simulink model "Tank_Modell_Student_R2013b"  (R2013a)
settings: Solver=ode45  StartTime=0.0  StopTime=400  MaxStep=1e-1  RelTol=1e-3
InitFcn:
  | set_parameter
StopFcn:
  | animation(h1_out,h2_out,q12_out,a1_out,a2_out,z1_out,anim_on,video_on);
values from neighbouring files (symbols this model uses):
  parInit =     [parameter_08.mat]
  parSys =     [parameter_08.mat]
undefined symbols (not defined in the file or in its folder): parSollwertfilter
libraries: simulink x3
settings Model: Creator=Wolfgang Kemmetmüller  LastModifiedBy=Christoph Zech
settings DataIOCC: SignalLoggingSaveFormat=ModelDataLogs
settings OptimizationCC: ExpressionDepthLimit=2147483647  InitFltsAndDblsToZero=on
settings DebuggingCC: SaveWithParameterizedLinksMsg=none  MultiTaskDSMMsg=warning  MultiTaskCondExecSysMsg=none  FrameProcessingCompatibilityMsg=error  StrictBusMsg=None
settings SFSimCC: SimParseCustomCode=off
settings RTWCC: IncludeERTFirstTime=on
settings GRTTargetCC: CodeReplacementLibrary=C89/C90 (ANSI)  CombineOutputUpdateFcns=off  GRTInterface=on

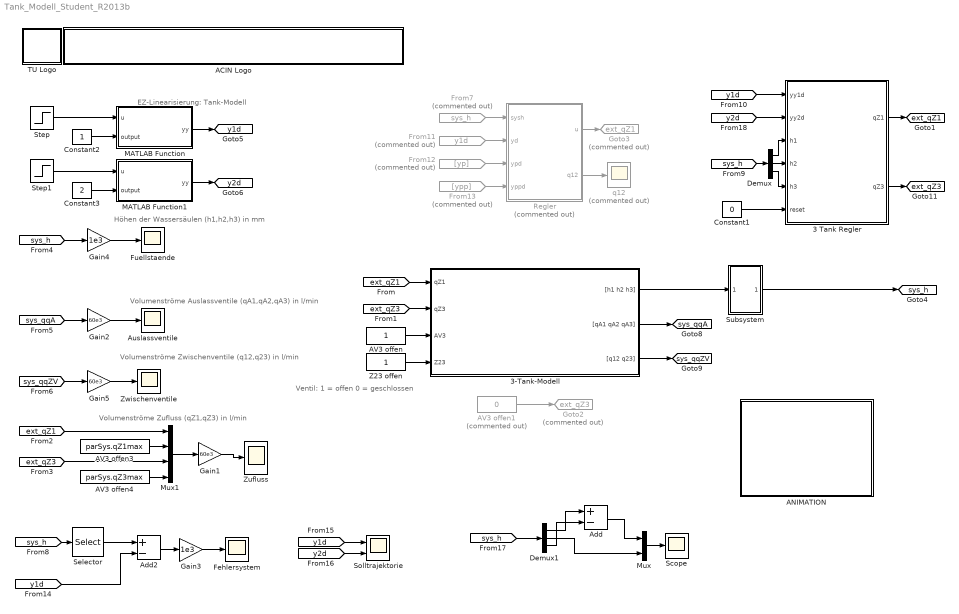
== system Tank_Modell_Student_R2013b ==
  note: EZ-Linearisierung: Tank-Modell
  note: Höhen der Wassersäulen (h1,h2,h3) in mm
  note: Volumenströme Auslassventile (qA1,qA2,qA3) in l/min
  note: Volumenströme Zwischenventile (q12,q23) in l/min
  note: Ventil:
      | 1 = offen
      | 0 = geschlossen
  note: Volumenströme Zufluss (qZ1,qZ3) in l/min
  3 Tank Regler : MATLAB Function  TreatAsAtomicUnit=on
  3-Tank-Modell : Subsystem
      mask init:
      | S = get_param(gcb,'UserData');
      mask Display:
      | image(S.pic);
      | port_label('input', 1, 'qZ1');
      | port_label('input', 2, 'qZ3');
      | port_label('input', 3, 'AV3');
      | port_label('input', 4, 'Z23');
      | port_label('output', 1, '[h1 h2 h3]');
      | port_label('output', 2, '[qA1 qA2 qA3]');
      | port_label('output', 3, '[q12 q23]');
  ACIN Logo : Subsystem
      mask init:
      | s = get_param(gcb,'UserData');
      mask Display:
      | image(s.logo,[0 0 439 45]);
      | %axis image
  ANIMATION : Subsystem
      mask init:
      | S = get_param(gcb,'UserData');
      mask Display: image(imread('Fisch.jpg'));
  AV3 offen : Constant
  AV3 offen1 : Constant  Commented=on  Value=0
  AV3 offen3 : Constant  Value=parSys.qZ1max  SampleTime=parSys.Ta
  AV3 offen4 : Constant  Value=parSys.qZ3max  SampleTime=parSys.Ta
  Add : Sum  Inputs=+-
  Add2 : Sum  Inputs=+-
  Auslassventile : Scope
      settings: ShowLegends=on  YMin=0.56181  YMax=1.40614
  Constant1 : Constant  Value=0
  Constant2 : Constant
  Constant3 : Constant  Value=2
  Demux : Demux  Outputs=3
  Demux1 : Demux  Outputs=3
  Fehlersystem : Scope
      settings: ShowLegends=on  YMin=-10  YMax=140  SaveName=ScopeData2
  From11 : From  Commented=on  GotoTag=y1d  TagVisibility=global
  From12 : From  Commented=on  GotoTag=yp  TagVisibility=global
  From13 : From  Commented=on  GotoTag=ypp  TagVisibility=global
  From7 : From  Commented=on  GotoTag=sys_h  TagVisibility=global
  Fuellstaende : Scope
      settings: ShowLegends=on  YMin=90  YMax=250
  Gain1 : Gain  Gain=60e3
  Gain2 : Gain  Gain=60e3
  Gain3 : Gain  Gain=1e3
  Gain4 : Gain  Gain=1e3
  Gain5 : Gain  Gain=60e3
  Goto2 : Goto  Commented=on  GotoTag=ext_qZ3  TagVisibility=global
  Goto3 : Goto  Commented=on  GotoTag=ext_qZ1  TagVisibility=global
  MATLAB Function : MATLAB Function  TreatAsAtomicUnit=on  SystemSampleTime=parSollwertfilter.Ta
  MATLAB Function1 : MATLAB Function  TreatAsAtomicUnit=on  SystemSampleTime=parSollwertfilter.Ta
  Mux : Mux  Inputs=2
  Mux1 : Mux
  "Regler " : MATLAB Function  Commented=on  TreatAsAtomicUnit=on
  Scope : Scope
      settings: YMin=0.03  YMax=0.21  SaveName=ScopeData5
  Selector : Selector  InputPortWidth=3  IndexOptions=Index vector (dialog)  Indices=[2]  OutputSizes=1
  Solltrajektorie : Scope  NumInputPorts=2
      settings: YMin=-0.0125~-0.0125  YMax=0.1125~0.1125
  Step : Step  Before=parSys.h2_0  After=parSys.h2_0+0.1  SampleTime=0
  Step1 : Step  Before=parSys.h1_0-parSys.h3_0  After=parSys.h1_0-parSys.h3_0-0.05  SampleTime=0
  Subsystem : Subsystem
  TU Logo : Subsystem
      mask init:
      | s = get_param(gcb,'UserData');
      mask Display: image(s.logo,[0 0 45 45]);
  Z23 offen : Constant
  Zufluss : Scope
      settings: ShowLegends=on  YMin=-7.5  YMax=22.5  SaveName=ScopeData3
  Zwischenventile : Scope
      settings: YMin=-10  YMax=10  SaveName=ScopeData2
  q12 : Scope  Commented=on
      settings: ShowLegends=on  YMin=0.000014  YMax=0.000028  SaveName=ScopeData4
  tag scope: ext_qZ1=global, ext_qZ3=global, sys_h=global, sys_qqA=global, sys_qqZV=global, y1d=global, y2d=global
  wires:
  [sys_qqA] -> Gain2/1
  [sys_qqZV] -> Gain5/1
  [sys_h] -> Gain4/1
  3-Tank-Modell/3("[q12 q23]") -> [sys_qqZV]
  3-Tank-Modell/2("[qA1 qA2 qA3]") -> [sys_qqA]
  AV3 offen/1 -> 3-Tank-Modell/3(AV3)
  Z23 offen/1 -> 3-Tank-Modell/4(Z23)
  [ext_qZ1] -> 3-Tank-Modell/1(qZ1)
  [ext_qZ3] -> 3-Tank-Modell/2(qZ3)
  [ext_qZ1] -> Mux1/1
  [ext_qZ3] -> Mux1/3
  AV3 offen3/1 -> Mux1/2
  AV3 offen4/1 -> Mux1/4
  Gain5/1 -> Zwischenventile/1
  Gain2/1 -> Auslassventile/1
  Gain4/1 -> Fuellstaende/1
  Mux1/1 -> Gain1/1
  Gain1/1 -> Zufluss/1
  AV3 offen1/1 -> Goto2/1
  "Regler "/1(u) -> Goto3/1
  From7/1 -> "Regler "/1(sysh)
  [sys_h] -> Selector/1
  Selector/1 -> Add2/1
  "Regler "/2(q12) -> q12/1
  MATLAB Function/1(yy) -> [y1d]
  From11/1 -> "Regler "/2(yd)
  From12/1 -> "Regler "/3(ypd)
  From13/1 -> "Regler "/4(yppd)
  [y1d] -> Add2/2
  [y1d] -> Solltrajektorie/1
  [y2d] -> Solltrajektorie/2
  Add2/1 -> Gain3/1
  Gain3/1 -> Fehlersystem/1
  [sys_h] -> Demux/1
  Demux/1 -> 3 Tank Regler/3(h1)
  Demux/2 -> 3 Tank Regler/4(h2)
  Demux/3 -> 3 Tank Regler/5(h3)
  3 Tank Regler/1(qZ1) -> [ext_qZ1]
  3 Tank Regler/2(qZ3) -> [ext_qZ3]
  Constant1/1 -> 3 Tank Regler/6(reset)
  [y1d] -> 3 Tank Regler/1(yy1d)
  Constant2/1 -> MATLAB Function/2(output)
  MATLAB Function1/1(yy) -> [y2d]
  Constant3/1 -> MATLAB Function1/2(output)
  [y2d] -> 3 Tank Regler/2(yy2d)
  Step/1 -> MATLAB Function/1(u)
  Step1/1 -> MATLAB Function1/1(u)
  [sys_h] -> Demux1/1
  Demux1/1 -> Add/1
  Demux1/3 -> Add/2
  Mux/1 -> Scope/1
  Add/1 -> Mux/1
  Demux1/2 -> Mux/2
  3-Tank-Modell/1("[h1 h2 h3]") -> Subsystem/1(In1)
  Subsystem/1(Out1) -> [sys_h]

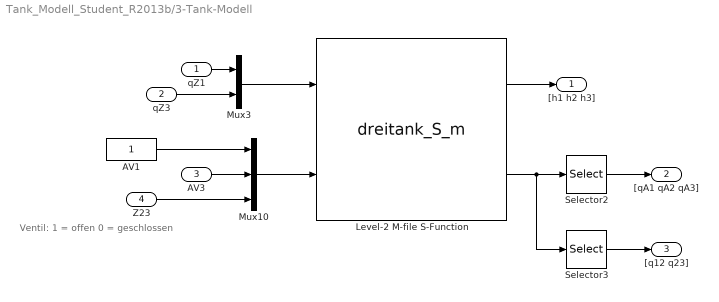
== system Tank_Modell_Student_R2013b/3-Tank-Modell ==
  note: Ventil:
      | 1 = offen
      | 0 = geschlossen
  qZ1 : Inport
  qZ3 : Inport  Port=2
  AV3 : Inport  Port=3
  Z23 : Inport  Port=4
  AV1 : Constant
  Level-2 M-file S-Function : M-S-Function  FunctionName=dreitank_S_m  Parameters=Atank, rho, eta, g, alphaA1, DA1, alphaA2, A2, alphaA3, DA3, alpha12_0, A12, Dh12, lambdac12, alpha23_0, D23, lambdac23, hmin, h1_0, h2_0, h3_0, qZ1max, qZ3max, flaglimqZ, h_max, h_min  mask{Atank=parSys.Atank, rho=parSys.rho, eta=parSys.eta, g=parSys.g, alphaA1=parSys.alphaA1, DA1=parSys.DA1, alphaA2=parSys.alphaA2, A2=parSys.A2, alphaA3=parSys.alphaA3, DA3=parSys.DA3, alpha12_0=parSys.alpha12_0, A12=parSys.A12, Dh12=parSys.Dh12, lambdac12=parSys.lambdac12, alpha23_0=parSys.alpha23_0, D23=parSys.D23, lambdac23=parSys.lambdac23, hmin=parSys.hmin, h1_0=parSys.h1_0, h2_0=parSys.h2_0, h3_0=parSys.h3_0, qZ1max=parSys.qZ1max, qZ3max=parSys.qZ3max, h_max=parSys.hmax, h_min=parSys.hmin, flaglimqZ=off}
      mask prompts: Atank "Grundfläche Tank (Atank)"; rho "Dichte Wasser (rho)"; eta "Viskosität Wasser (eta)"; g "Gravitationskonstante (g)"; alphaA1 "Kontraktionskoeffizient AV1 (alphaA1)"; DA1 "Durchmesser AV1 (DA1)"; alphaA2 "Kontraktionskoeffizient AV2 (alphaA2)"; A2 "Querschnittsfläche AV2 (A2)"; alphaA3 "Kontraktionskoeffizient AV3 (alphaA3)"; DA3 "Durchmesser A3 (DA3)"; alpha12_0 "Kontraktionskoeffizient ZV12 (alpha12_0)"; A12 "Querschnittsfläche ZV12 (A12)"; Dh12 "hydraulischer Durchmesser ZV12 (Dh12)"; lambdac12 "kritische Fließzahl ZV12 (lambdac12)"; alpha23_0 "Kontraktionskoeffizient ZV23 (alpha23_0)"; D23 "Durchmesser ZV23 (D23)"; lambdac23 "kritische Fließzahl ZV23 (lambdac23)"; hmin "minimale Füllhöhe (hmin)"; h1_0 "Anfangsbedingung h1 (h1_0)"; h2_0 "Anfangsbedingung h2 (h2_0)"; h3_0 "Anfangsbedingung h3 (h3_0)"; qZ1max "maximaler Zufluss Z1 (qZ1max)"; qZ3max "maximaler Zufluss Z3 (qZ3max)"; h_max "Maximale Füllhöhe"; h_min "Minimale Füllhöhe"; flaglimqZ "Beschränkung der Zuflüsse ein"
      mask Display:
      | port_label('input',1,'Zulaufvolumenströme')
      | port_label('input',2,'Zustand Ventile')
      | 
      | port_label('output',1,'Zustände')
      | port_label('output',2,'Volumenströme')
  Mux10 : Mux  Inputs=3
  Mux3 : Mux  Inputs=2
  Selector2 : Selector  InputPortWidth=5  IndexOptions=Index vector (dialog)  Indices=[1 2 3]  OutputSizes=1
  Selector3 : Selector  InputPortWidth=5  IndexOptions=Index vector (dialog)  Indices=[4 5]  OutputSizes=1
  "[h1 h2 h3]" : Outport
  "[qA1 qA2 qA3]" : Outport  Port=2
  "[q12 q23]" : Outport  Port=3
  wires:
  AV1/1 -> Mux10/1
  Mux3/1 -> Level-2 M-file S-Function/1
  Mux10/1 -> Level-2 M-file S-Function/2
  qZ1/1 -> Mux3/1
  Level-2 M-file S-Function/1 -> "[h1 h2 h3]"/1
  qZ3/1 -> Mux3/2
  Level-2 M-file S-Function/2 -> Selector2/1, Selector3/1
  Selector2/1 -> "[qA1 qA2 qA3]"/1
  Selector3/1 -> "[q12 q23]"/1
  Z23/1 -> Mux10/3
  AV3/1 -> Mux10/2

== system Tank_Modell_Student_R2013b/ACIN Logo ==

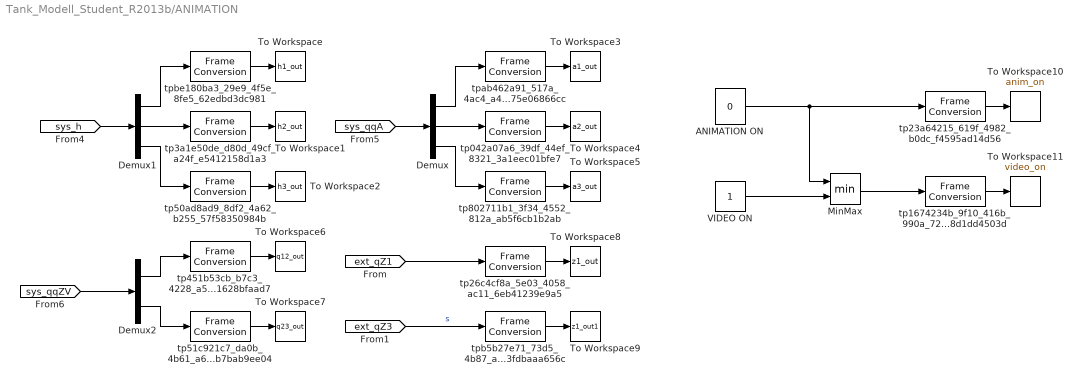
== system Tank_Modell_Student_R2013b/ANIMATION ==
  ANIMATION ON : Constant  Value=0
  Demux : Demux  Outputs=3
  Demux1 : Demux  Outputs=3
  Demux2 : Demux  Outputs=2
  MinMax : MinMax  Inputs=2
  To Workspace : ToWorkspace  VariableName=h1_out  SampleTime=parSys.Ta
  To Workspace1 : ToWorkspace  VariableName=h2_out  SampleTime=parSys.Ta
  To Workspace10 : ToWorkspace  VariableName=anim_on  SampleTime=50
  To Workspace11 : ToWorkspace  VariableName=video_on  SampleTime=50
  To Workspace2 : ToWorkspace  VariableName=h3_out  SampleTime=parSys.Ta
  To Workspace3 : ToWorkspace  VariableName=a1_out  SampleTime=parSys.Ta
  To Workspace4 : ToWorkspace  VariableName=a2_out  SampleTime=parSys.Ta
  To Workspace5 : ToWorkspace  VariableName=a3_out  SampleTime=parSys.Ta
  To Workspace6 : ToWorkspace  VariableName=q12_out  SampleTime=parSys.Ta
  To Workspace7 : ToWorkspace  VariableName=q23_out  SampleTime=parSys.Ta
  To Workspace8 : ToWorkspace  VariableName=z1_out  SampleTime=parSys.Ta
  To Workspace9 : ToWorkspace  VariableName=z1_out1  SampleTime=parSys.Ta
  VIDEO ON : Constant
  tp042a07a6_39df_44ef_8321_3a1eec01bfe7 : FrameConversion  OutFrame=Sample-based
  tp1674234b_9f10_416b_990a_728d1dd4503d : FrameConversion  OutFrame=Sample-based
  tp23a64215_619f_4982_b0dc_f4595ad14d56 : FrameConversion  OutFrame=Sample-based
  tp26c4cf8a_5e03_4058_ac11_6eb41239e9a5 : FrameConversion  OutFrame=Sample-based
  tp3a1e50de_d80d_49cf_a24f_e5412158d1a3 : FrameConversion  OutFrame=Sample-based
  tp451b53cb_b7c3_4228_a556_c61628bfaad7 : FrameConversion  OutFrame=Sample-based
  tp50ad8ad9_8df2_4a62_b255_57f58350984b : FrameConversion  OutFrame=Sample-based
  tp51c921c7_da0b_4b61_a6ab_b6b7bab9ee04 : FrameConversion  OutFrame=Sample-based
  tp802711b1_3f34_4552_812a_ab5f6cb1b2ab : FrameConversion  OutFrame=Sample-based
  tpab462a91_517a_4ac4_a466_6d75e06866cc : FrameConversion  OutFrame=Sample-based
  tpb5b27e71_73d5_4b87_ab88_53fdbaaa656c : FrameConversion  OutFrame=Sample-based
  tpbe180ba3_29e9_4f5e_8fe5_62edbd3dc981 : FrameConversion  OutFrame=Sample-based
  wires:
  [sys_qqA] -> Demux/1
  [sys_h] -> Demux1/1
  [sys_qqZV] -> Demux2/1
  ANIMATION ON/1 -> MinMax/1, tp23a64215_619f_4982_b0dc_f4595ad14d56/1
  VIDEO ON/1 -> MinMax/2
  Demux1/1 -> tpbe180ba3_29e9_4f5e_8fe5_62edbd3dc981/1
  tpbe180ba3_29e9_4f5e_8fe5_62edbd3dc981/1 -> To Workspace/1
  Demux1/2 -> tp3a1e50de_d80d_49cf_a24f_e5412158d1a3/1
  tp3a1e50de_d80d_49cf_a24f_e5412158d1a3/1 -> To Workspace1/1
  tp23a64215_619f_4982_b0dc_f4595ad14d56/1 -> To Workspace10/1
  MinMax/1 -> tp1674234b_9f10_416b_990a_728d1dd4503d/1
  tp1674234b_9f10_416b_990a_728d1dd4503d/1 -> To Workspace11/1
  Demux1/3 -> tp50ad8ad9_8df2_4a62_b255_57f58350984b/1
  tp50ad8ad9_8df2_4a62_b255_57f58350984b/1 -> To Workspace2/1
  Demux/1 -> tpab462a91_517a_4ac4_a466_6d75e06866cc/1
  tpab462a91_517a_4ac4_a466_6d75e06866cc/1 -> To Workspace3/1
  Demux/2 -> tp042a07a6_39df_44ef_8321_3a1eec01bfe7/1
  tp042a07a6_39df_44ef_8321_3a1eec01bfe7/1 -> To Workspace4/1
  Demux/3 -> tp802711b1_3f34_4552_812a_ab5f6cb1b2ab/1
  tp802711b1_3f34_4552_812a_ab5f6cb1b2ab/1 -> To Workspace5/1
  Demux2/1 -> tp451b53cb_b7c3_4228_a556_c61628bfaad7/1
  tp451b53cb_b7c3_4228_a556_c61628bfaad7/1 -> To Workspace6/1
  Demux2/2 -> tp51c921c7_da0b_4b61_a6ab_b6b7bab9ee04/1
  tp51c921c7_da0b_4b61_a6ab_b6b7bab9ee04/1 -> To Workspace7/1
  [ext_qZ1] -> tp26c4cf8a_5e03_4058_ac11_6eb41239e9a5/1
  tp26c4cf8a_5e03_4058_ac11_6eb41239e9a5/1 -> To Workspace8/1
  [ext_qZ3] -> tpb5b27e71_73d5_4b87_ab88_53fdbaaa656c/1  "s"
  tpb5b27e71_73d5_4b87_ab88_53fdbaaa656c/1 -> To Workspace9/1

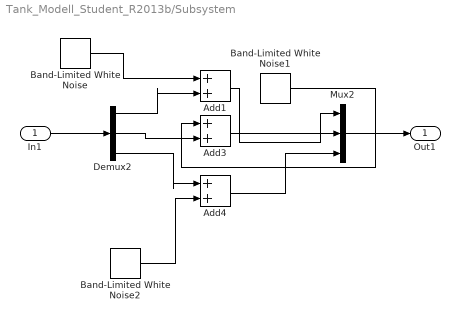
== system Tank_Modell_Student_R2013b/Subsystem ==
  In1 : Inport
  Add1 : Sum
  Add3 : Sum
  Add4 : Sum
  Band-Limited White Noise : simulink/Sources/Band-Limited White Noise  Cov=[25e-10]  Ts=0.1  seed=[23341]
  Band-Limited White Noise1 : simulink/Sources/Band-Limited White Noise  Cov=[25e-10]  Ts=0.1  seed=[93754]
  Band-Limited White Noise2 : simulink/Sources/Band-Limited White Noise  Cov=[25e-10]  Ts=0.1  seed=[35936]
  Demux2 : Demux  Outputs=3
  Mux2 : Mux  Inputs=3
  Out1 : Outport
  wires:
  Mux2/1 -> Out1/1
  In1/1 -> Demux2/1
  Add4/1 -> Mux2/3
  Demux2/2 -> Add3/2
  Band-Limited White Noise2/1 -> Add4/2
  Band-Limited White Noise1/1 -> Add3/1
  Demux2/3 -> Add4/1
  Demux2/1 -> Add1/2
  Band-Limited White Noise/1 -> Add1/1
  Add1/1 -> Mux2/1
  Add3/1 -> Mux2/2

== system Tank_Modell_Student_R2013b/TU Logo ==

== matlab function Tank_Modell_Student_R2013b/MATLAB Function ==
  settings: updateMethod=DISCRETE  sampleTime=parSollwertfilter.Ta
  data: u input; output input; yy output; parSollwertfilter parameter; parSys parameter
function yy  = sollwertfilter(u, output, parSollwertfilter, parSys)
persistent x;

if output < 1.5
    u = u-parSys.h2_0; % Anfangswert abziehen
else
    u = u-parSys.h1_0+parSys.h3_0;
end

a=parSollwertfilter.a;
b=parSollwertfilter.b;
c=parSollwertfilter.c;
d=parSollwertfilter.d;

if(isempty(x))
    x0_Filter=parSollwertfilter.x0_Filter;
    x=x0_Filter;
end

yt=c*x+d*u;

if output < 1.5
    y=yt(1)+parSys.h2_0; % Anfangswert wieder addieren
else
    y=yt(1)+parSys.h1_0-parSys.h3_0; % Anfangswert wieder addieren
end
yp=yt(2);
ypp=yt(3);

yy = [y; yp; ypp];

x=a*x+b*u;

== matlab function Tank_Modell_Student_R2013b/Regler  ==
  settings: updateMethod=DISCRETE  sampleTime=parSys.Ta
  data: u output; sysh input; parSys parameter; yd input; ypd input; yppd input; q12 output
function [u,q12]  = fcn(sysh, parSys, yd, ypd, yppd)

Atank = parSys.Atank;
rho = parSys.rho;
eta = parSys.eta;
g = parSys.g;
alphaA1 = parSys.alphaA1;
DA1 = parSys.DA1;
alphaA2 = parSys.alphaA2;
A2 = parSys.A2;
alphaA3 = parSys.alphaA3;
DA3 = parSys.DA3;
alpha12_0 = parSys.alpha12_0;
A12 = parSys.A12;
Dh12 = parSys.Dh12;
lambdac12 = parSys.lambdac12;
alpha23_0 = parSys.alpha23_0;
D23 = parSys.D23;
lambdac23 = parSys.lambdac23;
hmin = parSys.hmin;
hmax = parSys.hmax;
dh12min = parSys.dh12min;
a0 = parSys.a0;
a1 = parSys.a1;

h1=sysh(1);
h2=sysh(2);
qA1 = alphaA1 * DA1 ^ 2 * pi * sqrt(0.2e1) * sqrt(g) * sqrt(h1) / 0.4e1;
qA2 = alphaA2 * A2 * sqrt(0.2e1) * sqrt(g) * sqrt(h2);

dqA2_dh2 = alphaA2 * A2 * sqrt(0.2e1) * sqrt(g) * h2 ^ (-0.1e1 / 0.2e1) / 0.2e1;

if abs(h1-h2) > dh12min
    dq12_dh1 = 0.2e1 * alpha12_0 * Dh12 * rho / eta * g / lambdac12 * (0.1e1 - tanh(0.2e1 * Dh12 * rho / eta * sqrt(0.2e1) * sqrt(g) * sqrt(abs(h1 - h2)) / lambdac12) ^ 2) * A12 + alpha12_0 * tanh(0.2e1 * Dh12 * rho / eta * sqrt(0.2e1) * sqrt(g) * sqrt(abs(h1 - h2)) / lambdac12) * A12 * sqrt(0.2e1) * sqrt(g) * (abs(h1 - h2) ^ (-0.1e1 / 0.2e1)) / 0.2e1;
    dq12_dh2 = -0.2e1 * alpha12_0 * Dh12 * rho / eta * g / lambdac12 * (0.1e1 - tanh(0.2e1 * Dh12 * rho / eta * sqrt(0.2e1) * sqrt(g) * sqrt(abs(h1 - h2)) / lambdac12) ^ 2) * A12 - alpha12_0 * tanh(0.2e1 * Dh12 * rho / eta * sqrt(0.2e1) * sqrt(g) * sqrt(abs(h1 - h2)) / lambdac12) * A12 * sqrt(0.2e1) * sqrt(g) * (abs(h1 - h2) ^ (-0.1e1 / 0.2e1)) / 0.2e1;
else
    %Linearisierung
    dq12_dh1 = parSys.d_dh1 + parSys.k_dh1*abs(h1-h2);
    dq12_dh2 = parSys.d_dh2 + parSys.k_dh2*abs(h1-h2);
end
q12 = alpha12_0 * tanh(0.2e1 * Dh12 * rho / eta * sqrt(0.2e1) * sqrt(g) * sqrt(abs(h1 - h2)) / lambdac12) * A12 * sqrt(0.2e1) * sqrt(g) * sqrt(abs(h1 - h2)) * sign((h1 - h2));

u = 0.1e1 / dq12_dh1 * Atank ^ 2 * (yppd - dq12_dh1 / Atank ^ 2 * (-q12 - qA1) - (dq12_dh2 - dqA2_dh2) / Atank ^ 2 * (q12 - qA2) - a0 * (h2 - yd) - a1 * ((q12 - qA2) / Atank - ypd));

== matlab function Tank_Modell_Student_R2013b/3 Tank Regler ==
  settings: updateMethod=DISCRETE  sampleTime=parSys.Ta
  data: qZ1 output; qZ3 output; yy1d input; yy2d input; h1 input; h2 input; h3 input; reset input; parSys parameter; parInit parameter
function [qZ1,qZ3]  = fcn(yy1d, yy2d, h1, h2, h3, reset, parSys, parInit)

persistent e1I;
persistent e2I;

if (isempty(e1I))
    e1I = 0;
end
if (isempty(e2I))
    e2I = 0;
end
if reset
    qZ1 = 0;
    qZ3 = 0;
    return
end
    

Atank = parSys.Atank;
rho = parSys.rho;
eta = parSys.eta;
g = parSys.g;
alphaA1 = parSys.alphaA1;
DA1 = parSys.DA1;
alphaA2 = parSys.alphaA2;
A2 = parSys.A2;
alphaA3 = parSys.alphaA3;
DA3 = parSys.DA3;
alpha12_0 = parSys.alpha12_0;
A12 = parSys.A12;
Dh12 = parSys.Dh12;
lambdac12 = parSys.lambdac12;
alpha23_0 = parSys.alpha23_0;
D23 = parSys.D23;
lambdac23 = parSys.lambdac23;
hmin = parSys.hmin;
hmax = parSys.hmax;
dh12min = parSys.dh12min;
a0 = parInit.a0;
a1 = parInit.a1;
dh23min = parSys.dh12min;

A3 = DA3^2*pi/4;
%laut angabe
Dh23 = D23;
A23 = D23^2*pi/4;

y1dpp = yy1d(3);
y1dp  = yy1d(2);
y1d   = yy1d(1);

y2dp  = yy2d(2);
y2d   = yy2d(1);


qA1 = alphaA1 * DA1 ^ 2 * pi * sqrt(0.2e1) * sqrt(g) * sqrt(h1) / 0.4e1;
qA2 = alphaA2 * A2 * sqrt(0.2e1) * sqrt(g) * sqrt(h2);
qA3 = alphaA3 * A3 * sqrt(0.2e1) * sqrt(g) * sqrt(h3);


dqA2_dh2 = alphaA2 * A2 * sqrt(0.2e1) * sqrt(g) * h2 ^ (-0.1e1 / 0.2e1) / 0.2e1;

if abs(h1-h2) > dh12min
    dq12_dh1 = 0.2e1 * alpha12_0 * Dh12 * rho / eta * g / lambdac12 * (0.1e1 - tanh(0.2e1 * Dh12 * rho / eta * sqrt(0.2e1) * sqrt(g) * sqrt(abs(h1 - h2)) / lambdac12) ^ 2) * A12 + alpha12_0 * tanh(0.2e1 * Dh12 * rho / eta * sqrt(0.2e1) * sqrt(g) * sqrt(abs(h1 - h2)) / lambdac12) * A12 * sqrt(0.2e1) * sqrt(g) * (abs(h1 - h2) ^ (-0.1e1 / 0.2e1)) / 0.2e1;
    dq12_dh2 = -0.2e1 * alpha12_0 * Dh12 * rho / eta * g / lambdac12 * (0.1e1 - tanh(0.2e1 * Dh12 * rho / eta * sqrt(0.2e1) * sqrt(g) * sqrt(abs(h1 - h2)) / lambdac12) ^ 2) * A12 - alpha12_0 * tanh(0.2e1 * Dh12 * rho / eta * sqrt(0.2e1) * sqrt(g) * sqrt(abs(h1 - h2)) / lambdac12) * A12 * sqrt(0.2e1) * sqrt(g) * (abs(h1 - h2) ^ (-0.1e1 / 0.2e1)) / 0.2e1;
else
    %Linearisierung
    dq12_dh1 = parSys.d_dq12_dh1 + parSys.k_dq12_dh1*abs(h1-h2);
    dq12_dh2 = parSys.d_dq12_dh2 + parSys.k_dq12_dh2*abs(h1-h2);
end

if abs(h2-h3) > dh23min
    dq23_dh2 = 0.2e1 * alpha23_0 * (0.1e1 - tanh(0.2e1 * Dh23 * rho / eta * sqrt(0.2e1) * sqrt(g) * sqrt(abs(h2 - h3)) / lambdac23) ^ 2) * Dh23 * rho / eta * g / lambdac23 * A23 + alpha23_0 * tanh(0.2e1 * Dh23 * rho / eta * sqrt(0.2e1) * sqrt(g) * sqrt(abs(h2 - h3)) / lambdac23) * A23 * sqrt(0.2e1) * sqrt(g) * (abs(h2 - h3)) ^ (-0.1e1 / 0.2e1) / 0.2e1;
    %dq23_dh3 = 0.2e1 * alpha23_0 * (0.1e1 - tanh(0.2e1 * Dh23 * rho / eta * sqrt(0.2e1) * sqrt(g) * sqrt(abs(h3 - h2)) / lambdac23) ^ 2) * Dh23 * rho / eta * g / lambdac23 * A23 + alpha23_0 * tanh(0.2e1 * Dh23 * rho / eta * sqrt(0.2e1) * sqrt(g) * sqrt(abs(h3 - h2)) / lambdac23) * A23 * sqrt(0.2e1) * sqrt(g) * (abs(h3 - h2)) ^ (-0.1e1 / 0.2e1) / 0.2e1;
    %dq23_dh3 = 0.2e1 * alpha23_0 * (0.1e1 - tanh(0.2e1 * Dh23 * rho / eta * sqrt(0.2e1) * sqrt(g) * sqrt(abs(h3 - h2)) / lambdac23) ^ 2) * Dh23 * rho / eta * g / lambdac23 * A23 - alpha23_0 * tanh(0.2e1 * Dh23 * rho / eta * sqrt(0.2e1) * sqrt(g) * sqrt(abs(h3 - h2)) / lambdac23) * A23 * sqrt(0.2e1) * sqrt(g) * (abs(h3 - h2)) ^ (-0.1e1 / 0.2e1) / 0.2e1;
    dq23_dh3 = -0.2e1 * alpha23_0 * (0.1e1 - tanh(0.2e1 * Dh23 * rho / eta * sqrt(0.2e1) * sqrt(g) * sqrt(abs(h2 - h3)) / lambdac23) ^ 2) * Dh23 * rho / eta * g / lambdac23 * A23 - alpha23_0 * tanh(0.2e1 * Dh23 * rho / eta * sqrt(0.2e1) * sqrt(g) * sqrt(abs(h2 - h3)) / lambdac23) * A23 * sqrt(0.2e1) * sqrt(g) * abs(h2 - h3) ^ (-0.1e1 / 0.2e1) / 0.2e1;
else
    %Linearisierung
    dq23_dh2 = parSys.d_dq23_dh2 + parSys.k_dq23_dh2*abs(h2-h3);
    dq23_dh3 = parSys.d_dq23_dh3 + parSys.k_dq23_dh3*abs(h2-h3);
end

q12 = alpha12_0 * tanh(0.2e1 * Dh12 * rho / eta * sqrt(0.2e1) * sqrt(g) * sqrt(abs(h1 - h2)) / lambdac12) * A12 * sqrt(0.2e1) * sqrt(g) * sqrt(abs(h1 - h2)) * sign((h1 - h2));
q23 = alpha23_0 * tanh(0.2e1 * Dh23 * rho / eta * sqrt(0.2e1) * sqrt(g) * sqrt(abs(h2 - h3)) / lambdac23) * A23 * sqrt(0.2e1) * sqrt(g) * sqrt(abs(h2 - h3)) * sign(h2 - h3);

Lfh1 = [(q12 - q23 - qA2) / Atank];
Lf2h1 = [dq12_dh1 / Atank ^ 2 * (-q12 - qA1) - dq23_dh2 / Atank ^ 2 * (q12 - q23 - qA2) - dq23_dh3 / Atank ^ 2 * (q23 - qA3)];
Lfh2 = [(-q12 - qA1) / Atank - (q23 - qA3) / Atank];
Lg2h2 = [-0.1e1 / Atank];
Lg1h2 = [0.1e1 / Atank];
Lg2Lf1h1 = [-dq23_dh3 / Atank ^ 2];
Lg1Lf1h1 = [dq12_dh1 / Atank ^ 2];


e1I = e1I + (h2-y1d);
e2I = e2I + (h1-h3-y2d);
v = [y1dpp - parInit.a10 * (h2 - y1d) - parInit.a11 * (Lfh1 - y1dp) - parInit.a1I*e1I;
     y2dp  - parInit.a20 * (h1 - h3 - y2d) - parInit.a2I*e2I
     ];

bb = [Lf2h1;Lfh2];
D_inv = [-Lg2h2 / (Lg1h2 * Lg2Lf1h1 - Lg2h2 * Lg1Lf1h1) Lg2Lf1h1 / (Lg1h2 * Lg2Lf1h1 - Lg2h2 * Lg1Lf1h1); Lg1h2 / (Lg1h2 * Lg2Lf1h1 - Lg2h2 * Lg1Lf1h1) -Lg1Lf1h1 / (Lg1h2 * Lg2Lf1h1 - Lg2h2 * Lg1Lf1h1);];
u_temp = D_inv*(-bb+v);
qZ1 = u_temp(1);
qZ3 = u_temp(2);
end

== matlab function Tank_Modell_Student_R2013b/MATLAB Function1 ==
  settings: updateMethod=DISCRETE  sampleTime=parSollwertfilter.Ta
  data: u input; output input; yy output; parSollwertfilter parameter; parSys parameter
function yy  = sollwertfilter(u, output, parSollwertfilter, parSys)
persistent x;

if output < 1.5
    u = u-parSys.h2_0; % Anfangswert abziehen
else
    u = u-parSys.h1_0+parSys.h3_0;
end

a=parSollwertfilter.a;
b=parSollwertfilter.b;
c=parSollwertfilter.c;
d=parSollwertfilter.d;

if(isempty(x))
    x0_Filter=parSollwertfilter.x0_Filter;
    x=x0_Filter;
end

yt=c*x+d*u;

if output < 1.5
    y=yt(1)+parSys.h2_0; % Anfangswert wieder addieren
else
    y=yt(1)+parSys.h1_0-parSys.h3_0; % Anfangswert wieder addieren
end
yp=yt(2);
ypp=yt(3);

yy = [y; yp; ypp];

x=a*x+b*u;
